simulink model "q_5dof_wand_vr_sphere_collision_atia"  (Simulink 9.1)
settings: Solver=ode1  StartTime=0.0  StopTime=inf  FixedStep=0.001  RelTol=1e-3  EnableMultiTasking=on
values from neighbouring files (symbols this model uses):
  COM = zeros(1,size(V1,2))    [atia_centroid.m]
  fromSI = [1e3 1e3 1e3 180/pi 180/pi]    [setup_wand.m]
  K_CURR = 0.5 * [1 1 -1 -1 1 1]    [setup_wand.m]
  kd = [kd_x kd_y kd_z kd_yaw kd_roll]    [setup_wand.m]
  kp = [kp_x kp_y kp_z kp_yaw kp_roll]    [setup_wand.m]
  vo_c = [0 75 -75] * 1e-3    [setup_wand.m]
  wn_f = 150    [setup_wand.m]
  zeta_f = 1    [setup_wand.m]
undefined symbols (not defined in the file or in its folder): DiscIntNeverNeededParam, HIL, qc_get_step_size, V_CUBE_atia_wand, Visualization
libraries: quarc_library x12
(part 1 of 2)
settings Model: Creator=pmartin  LastModifiedBy=atn227  SimulationMode=external  ExtModeTrigDuration=5000
settings SolverCC: PositivePriorityOrder=on
settings DataIOCC: LimitDataPoints=on  SignalLoggingSaveFormat=ModelDataLogs
settings OptimizationCC: ExpressionDepthLimit=2147483647  LifeSpan=auto
settings DebuggingCC: SolverPrmCheckMsg=warning  FcnCallInpInsideContextMsg=warning  StateNameClashWarn=warning
settings RTWCC: SystemTargetFile=quarc_win64.tlc  TemplateMakefile=quarc_default_tmf  Description=QUARC Win64 Target
settings STFCustomTargetCC: TargetPreCompLibLocation=C:\PROGRA~3\QUARC\lib\2018a\win64\release  ConcurrentExecutionCompliant=on  SystemTargetFile=quarc_win64.tlc
settings GRTTargetCC: TargetPreCompLibLocation=C:\PROGRA~3\QUARC\lib\2018a\win64\release  ParMdlRefBuildCompliant=off  CompOptLevelCompliant=off  MatFileLogging=off  CPPClassGenCompliant=off  UseToolchainInfoCompliant=off  ExtMode=on  ExtModeMexFile=quarc_comm

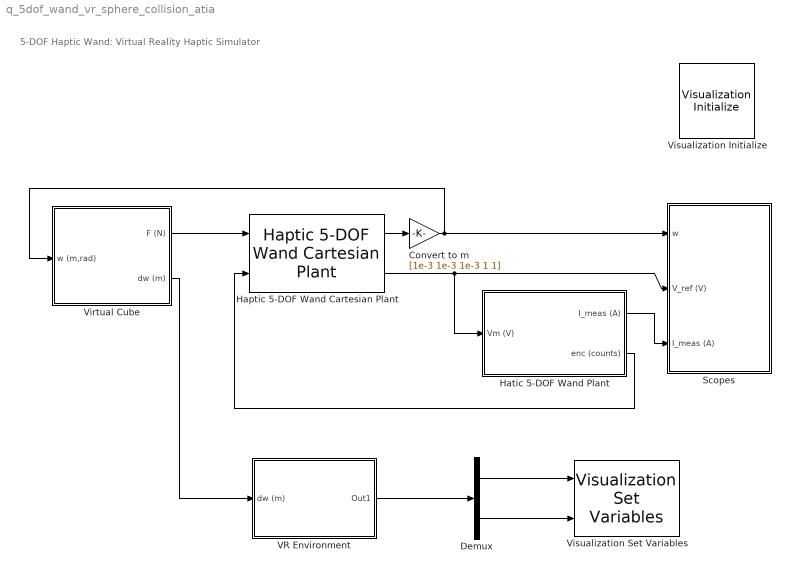
== system q_5dof_wand_vr_sphere_collision_atia ==
  note: 5-DOF Haptic Wand: Virtual Reality Haptic Simulator
  Convert to m : Gain  Gain=[1e-3 1e-3 1e-3 1 1]
  Demux : Demux  Outputs=2
  Haptic 5-DOF Wand Cartesian Plant : quarc_library/Devices/Quanser/Haptics/Pantographs/Haptic 5-DOF Wand/Interfacing/Haptic 5-DOF Wand Cartesian Plant
      settings: SourceProductName=QUARC Targets
  Hatic 5-DOF Wand Plant : Subsystem
  Scopes : Subsystem
  VR Environment : Subsystem
  Virtual Cube : Subsystem
  Visualization Initialize : quarc_library/User Interface/Visualization/Visualization Initialize  object_name=Visualization-1  scene_file=Visualization\5dof_wand_sphere.xml  uri={'normal','';'Configuration','shmem://%m:2';}  apply_uri_to_all_configs=off  server_send_size=1000000  server_receive_size=1000  derive_from_server=on  client_send_size=1000  client_receive_size=1000000  variables=[ 20 21 ]  initial_values=single([ 0 0 0 0 0 0 ])  open_on_start=on  close_on_stop=on
      settings: AttributesFormatString=%<object_name>  SourceProductName=QUARC Targets
  Visualization Set Variables : quarc_library/User Interface/Visualization/Visualization Set Variables  object_name=Visualization-1  offset=[ 3 0 ]  data_type=[ 0 0 ]  length=[ 3 3 ]  sample_time=visualization_get_frame_period  actor_name={'actor.cylinder/Orientation';'actor.cylinder/Position'}
      settings: AttributesFormatString=(%<object_name>)  SourceProductName=QUARC Targets
  wires:
  Virtual Cube/1(F (N)) -> Haptic 5-DOF Wand Cartesian Plant/1
  Virtual Cube/2(dw (m)) -> VR Environment/1(dw (m))
  Haptic 5-DOF Wand Cartesian Plant/2 -> Hatic 5-DOF Wand Plant/1(Vm (V)), Scopes/2(V_ref (V))
  Haptic 5-DOF Wand Cartesian Plant/1 -> Convert to m/1
  Convert to m/1 -> Scopes/1(w), Virtual Cube/1(w (m,rad))
  Hatic 5-DOF Wand Plant/1(I_meas (A)) -> Scopes/3(I_meas (A))
  Hatic 5-DOF Wand Plant/2(enc (counts)) -> Haptic 5-DOF Wand Cartesian Plant/2
  VR Environment/1(Out1) -> Demux/1
  Demux/2 -> Visualization Set Variables/2
  Demux/1 -> Visualization Set Variables/1

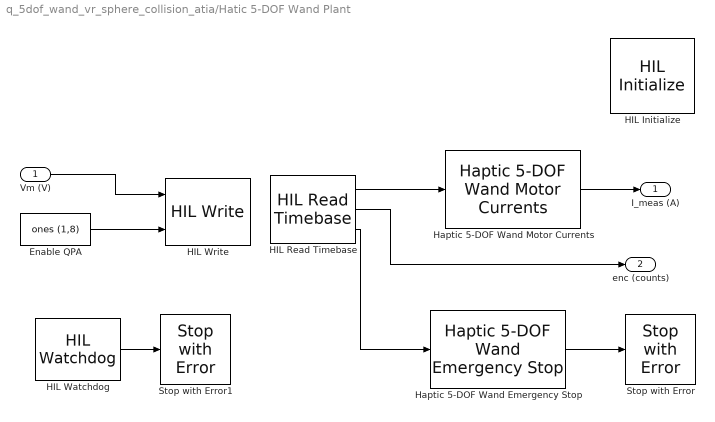
== system q_5dof_wand_vr_sphere_collision_atia/Hatic 5-DOF Wand Plant ==
  Vm (V) : Inport
  Enable QPA : Constant  Value=ones (1,8)
  HIL Initialize : quarc_library/Data Acquisition/Generic/Configuration/HIL Initialize  object_name=HIL-1  board_type=q8  board_number=0  board_options=""  exclusive=off  active=off  hardware_clocks=[0:1]  clock_modes=[0 0]  initial_clock_frequencies=[]  set_clock_params_at_start=on  set_clock_params_at_switch_in=off  set_clock_frequencies_at_start=off  set_clock_frequencies_at_switch_in=off  analog_input_channels=[0:7]  analog_input_configurations=[]  analog_input_maximums=10  analog_input_minimums=-10  set_analog_input_params_at_start=off  set_analog_input_params_at_switch_in=off  analog_output_channels=[0:7]  analog_output_maximums=[10]  analog_output_minimums=[-10]  initial_analog_outputs=[0]  final_analog_outputs=[0]  watchdog_analog_outputs=0  set_analog_output_params_at_start=on  set_analog_output_params_at_switch_in=off  set_analog_outputs_at_start=on  set_analog_outputs_at_switch_in=off  set_analog_outputs_at_terminate=on  set_analog_outputs_at_switch_out=off  set_analog_outputs_on_watchdog=off  digital_input_channels=[]  digital_output_channels=[]  digital_output_configuration=[]  initial_digital_outputs=[1]  final_digital_outputs=[1]  watchdog_digital_outputs=[2]  set_digital_output_params_at_start=off  set_digital_output_params_at_switch_in=off  set_digital_outputs_at_start=on  set_digital_outputs_at_switch_in=off  set_digital_outputs_at_terminate=on  set_digital_outputs_at_switch_out=off  set_digital_outputs_on_watchdog=off  encoder_channels=[0:7]  quadrature=[4]  encoder_filter_frequency=(1/120e-9)/1  initial_encoder_counts=[0]  set_encoder_params_at_start=on  set_encoder_params_at_switch_in=off  set_encoder_counts_at_start=on  set_encoder_counts_at_switch_in=off  pwm_channels=[]  pwm_modes=[0]  pwm_frequency=(1/60e-9)/1024  pwm_configuration=[]  pwm_alignment=[]  pwm_polarity=[]  pwm_leading_deadband=[]  pwm_trailing_deadband=[]  initial_pwm_outputs=[0]  final_pwm_outputs=[0]  watchdog_pwm_outputs=[]  set_pwm_params_at_start=on  set_pwm_params_at_switch_in=off  set_pwm_outputs_at_start=on  set_pwm_outputs_at_switch_in=off  set_pwm_outputs_at_terminate=on  set_pwm_outputs_at_switch_out=off  set_pwm_outputs_on_watchdog=off  other_output_channels=[]  initial_other_outputs=[]  final_other_outputs=[]  watchdog_other_outputs=[]  set_other_outputs_at_start=off  set_other_outputs_at_switch_in=off  set_other_outputs_at_terminate=off  set_other_outputs_at_switch_out=off  set_other_outputs_on_watchdog=off
  HIL Read Timebase : quarc_library/Data Acquisition/Generic/Timebases/HIL Read Timebase  object_name=HIL-1  clock=0  analog_channels=0:5  encoder_channels=[0:5]  digital_channels=[14,30]  other_channels=[]  samples_in_buffer=max(ceil(1/qc_get_step_size), 1)  active=on  vector_output=on  data_type_mode=Inherit via back propagation  encoder_data_type=double  digital_data_type=boolean
  HIL Watchdog : quarc_library/Data Acquisition/Generic/Watchdog/HIL Watchdog  object_name=HIL-1  timeout=qc_get_step_size*10  sample_time=qc_get_step_size  active=off
      settings: AttributesFormatString=(%<object_name>)  SourceProductName=QUARC Targets
  HIL Write : quarc_library/Data Acquisition/Generic/Immediate I//O/HIL Write  object_name=HIL-1  analog_channels=[0:5]  pwm_channels=[]  digital_channels=[0:3 16:19]  other_channels=[]  sample_time=-1  active=off  vector_input=on
  Haptic 5-DOF Wand Emergency Stop : quarc_library/Devices/Quanser/Haptics/Pantographs/Haptic 5-DOF Wand/Interfacing/Haptic 5-DOF Wand Emergency Stop
      settings: SourceProductName=QUARC Targets
  Haptic 5-DOF Wand Motor Currents : quarc_library/Devices/Quanser/Haptics/Pantographs/Haptic 5-DOF Wand/Interfacing/Haptic 5-DOF Wand Motor Currents
      settings: SourceProductName=QUARC Targets
  Stop with Error : quarc_library/Sinks/Error Handling/Stop with Error  message_type=Fixed error message  message=Controller Stopped - Emergency Stop Activated
      settings: AttributesFormatString="\"%<message>\""  SourceProductName=QUARC Targets
  Stop with Error1 : quarc_library/Sinks/Error Handling/Stop with Error  message_type=Fixed error message  message=Stopped by HIL Watchdog - Controller was running too slow
      settings: AttributesFormatString="\"%<message>\""  SourceProductName=QUARC Targets
  I_meas (A) : Outport
  enc (counts) : Outport  Port=2
  wires:
  Haptic 5-DOF Wand Emergency Stop/1 -> Stop with Error/1
  HIL Read Timebase/3 -> Haptic 5-DOF Wand Emergency Stop/1
  Haptic 5-DOF Wand Motor Currents/1 -> I_meas (A)/1
  HIL Read Timebase/2 -> enc (counts)/1
  HIL Read Timebase/1 -> Haptic 5-DOF Wand Motor Currents/1
  Enable QPA/1 -> HIL Write/2
  Vm (V)/1 -> HIL Write/1
  HIL Watchdog/1 -> Stop with Error1/1

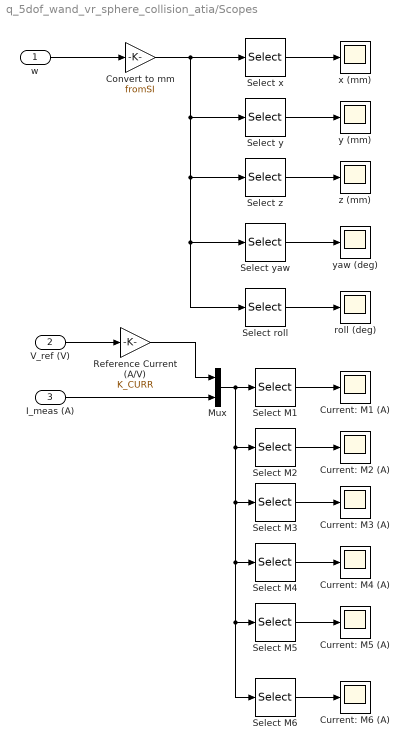
== system q_5dof_wand_vr_sphere_collision_atia/Scopes ==
  w : Inport
  V_ref (V) : Inport  Port=2
  I_meas (A) : Inport  Port=3
  Convert to mm : Gain  Gain=fromSI
  Current: M1 (A) : Scope
  Current: M2 (A) : Scope
  Current: M3 (A) : Scope
  Current: M4 (A) : Scope
  Current: M5 (A) : Scope
  Current: M6 (A) : Scope
  Mux : Mux  Inputs=2
  Reference Current (A/V) : Gain  Gain=K_CURR
  Select M1 : Selector  InputPortWidth=12  IndexOptions=Index vector (dialog)  Indices=[1 7]  OutputSizes=1
  Select M2 : Selector  InputPortWidth=12  IndexOptions=Index vector (dialog)  Indices=[2 8]  OutputSizes=1
  Select M3 : Selector  InputPortWidth=12  IndexOptions=Index vector (dialog)  Indices=[3 9]  OutputSizes=1
  Select M4 : Selector  InputPortWidth=12  IndexOptions=Index vector (dialog)  Indices=[4 10]  OutputSizes=1
  Select M5 : Selector  InputPortWidth=12  IndexOptions=Index vector (dialog)  Indices=[5 11]  OutputSizes=1
  Select M6 : Selector  InputPortWidth=12  IndexOptions=Index vector (dialog)  Indices=[6 12]  OutputSizes=1
  Select roll : Selector  InputPortWidth=5  IndexOptions=Index vector (dialog)  Indices=[5]  OutputSizes=1
  Select x : Selector  InputPortWidth=5  IndexOptions=Index vector (dialog)  Indices=[1]  OutputSizes=1
  Select y : Selector  InputPortWidth=5  IndexOptions=Index vector (dialog)  Indices=2  OutputSizes=1
  Select yaw : Selector  InputPortWidth=5  IndexOptions=Index vector (dialog)  Indices=4  OutputSizes=1
  Select z : Selector  InputPortWidth=5  IndexOptions=Index vector (dialog)  Indices=3  OutputSizes=1
  roll (deg) : Scope
  x (mm) : Scope
  y (mm) : Scope
  yaw (deg) : Scope
  z (mm) : Scope
  wires:
  Convert to mm/1 -> Select x/1, Select y/1, Select roll/1, Select yaw/1, Select z/1
  Select x/1 -> x (mm)/1
  w/1 -> Convert to mm/1
  Select y/1 -> y (mm)/1
  Select z/1 -> z (mm)/1
  Reference Current (A/V)/1 -> Mux/1
  I_meas (A)/1 -> Mux/2
  V_ref (V)/1 -> Reference Current (A/V)/1
  Select yaw/1 -> yaw (deg)/1
  Select roll/1 -> roll (deg)/1
  Mux/1 -> Select M1/1, Select M6/1, Select M5/1, Select M4/1, Select M3/1, Select M2/1
  Select M1/1 -> Current: M1 (A)/1
  Select M2/1 -> Current: M2 (A)/1
  Select M3/1 -> Current: M3 (A)/1
  Select M4/1 -> Current: M4 (A)/1
  Select M5/1 -> Current: M5 (A)/1
  Select M6/1 -> Current: M6 (A)/1

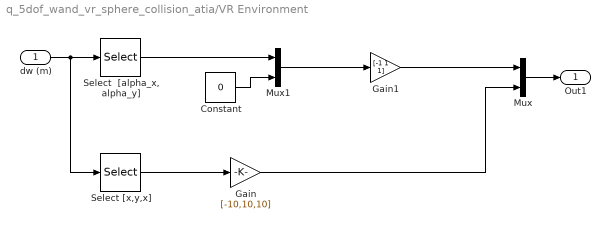
== system q_5dof_wand_vr_sphere_collision_atia/VR Environment ==
  dw (m) : Inport
  Constant : Constant  Value=0
  Gain : Gain  Gain=[-10,10,10]
  Gain1 : Gain  Gain=[-1 1 1]
  Mux : Mux  Inputs=2
  Mux1 : Mux  Inputs=2
  "Select  [alpha_x, alpha_y]" : Selector  InputPortWidth=5  IndexOptions=Index vector (dialog)  Indices=[5,4]  OutputSizes=1
  Select [x,y,x] : Selector  InputPortWidth=5  IndexOptions=Index vector (dialog)  Indices=[2 1 3]  OutputSizes=1
  Out1 : Outport
  wires:
  dw (m)/1 -> "Select  [alpha_x, alpha_y]"/1, Select [x,y,x]/1
  Select [x,y,x]/1 -> Gain/1
  Gain/1 -> Mux/2
  Mux/1 -> Out1/1
  "Select  [alpha_x, alpha_y]"/1 -> Mux1/1
  Mux1/1 -> Gain1/1
  Constant/1 -> Mux1/2
  Gain1/1 -> Mux/1

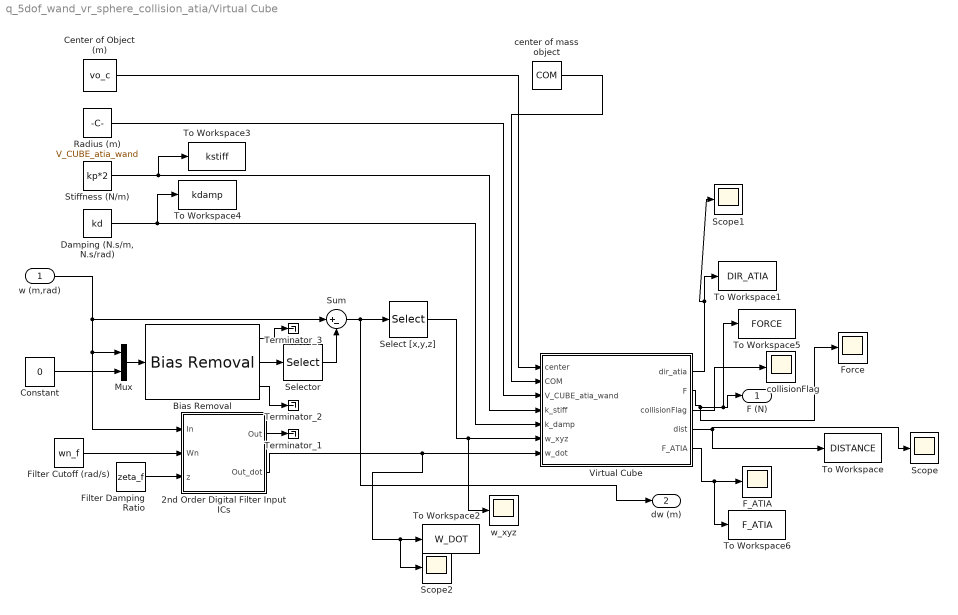
== system q_5dof_wand_vr_sphere_collision_atia/Virtual Cube ==
  w (m,rad) : Inport
  2nd Order Digital Filter Input ICs : Subsystem
  Bias Removal : quarc_library/Discrete/Bias Removal  start_time=0  end_time=qc_get_step_size  switch_id=0  sample_time=qc_get_step_size
      settings: SourceProductName=QUARC Targets
  Center of Object (m) : Constant  Value=vo_c
  Constant : Constant  Value=0
  "Damping (N.s/m, N.s/rad)" : Constant  Value=kd
  F_ATIA : Scope
  Filter Cutoff (rad/s) : Constant  Value=wn_f
  Filter Damping Ratio : Constant  Value=zeta_f
  Force : Scope
  Mux : Mux  Inputs=2
  Radius (m) : Constant  Value=V_CUBE_atia_wand
  Scope : Scope
  Scope1 : Scope
  Scope2 : Scope
  Select [x,y,z] : Selector  InputPortWidth=5  IndexOptions=Index vector (dialog)  Indices=1:3  OutputSizes=1
  Selector : Selector  InputPortWidth=6  IndexOptions=Index vector (dialog)  Indices=1:5  OutputSizes=1
  Stiffness (N/m) : Constant  Value=kp*2
  Sum : Sum  Inputs=|+-
  Terminator_1 : Terminator
  Terminator_2 : Terminator
  Terminator_3 : Terminator
  To Workspace : ToWorkspace  VariableName=DISTANCE  SaveFormat=Timeseries  SampleTime=-1
  To Workspace1 : ToWorkspace  VariableName=DIR_ATIA  SaveFormat=Timeseries  SampleTime=-1
  To Workspace2 : ToWorkspace  VariableName=W_DOT  SaveFormat=Timeseries  SampleTime=-1
      settings: Save2DSignal=2-D array (concatenate along first dimension)
  To Workspace3 : ToWorkspace  VariableName=kstiff  SampleTime=-1
      settings: Save2DSignal=2-D array (concatenate along first dimension)
  To Workspace4 : ToWorkspace  VariableName=kdamp  SampleTime=-1
      settings: Save2DSignal=2-D array (concatenate along first dimension)
  To Workspace5 : ToWorkspace  VariableName=FORCE  SaveFormat=Timeseries  SampleTime=-1
  To Workspace6 : ToWorkspace  VariableName=F_ATIA  SaveFormat=Timeseries  SampleTime=-1
  Virtual Cube : MATLAB Function  TreatAsAtomicUnit=on
  center of mass object : Constant  Value=COM
  collisionFlag : Scope
  w_xyz : Scope
  F (N) : Outport
  dw (m) : Outport  Port=2
  wires:
  Mux/1 -> Bias Removal/1
  Bias Removal/2 -> Selector/1
  Constant/1 -> Mux/2
  w (m,rad)/1 -> Sum/1, Mux/1, 2nd Order Digital Filter Input ICs/1(In)
  Radius (m)/1 -> Virtual Cube/3(V_CUBE_atia_wand)
  Sum/1 -> Select [x,y,z]/1, dw (m)/1
  Selector/1 -> Sum/2
  Center of Object (m)/1 -> Virtual Cube/1(center)
  Stiffness (N/m)/1 -> To Workspace3/1, Virtual Cube/4(k_stiff)
  "Damping (N.s/m, N.s/rad)"/1 -> To Workspace4/1, Virtual Cube/5(k_damp)
  Filter Cutoff (rad/s)/1 -> 2nd Order Digital Filter Input ICs/2(Wn)
  Filter Damping Ratio/1 -> 2nd Order Digital Filter Input ICs/3(z)
  2nd Order Digital Filter Input ICs/2(Out_dot) -> Scope2/1, To Workspace2/1, Virtual Cube/7(w_dot)
  2nd Order Digital Filter Input ICs/1(Out) -> Terminator_1/1
  Select [x,y,z]/1 -> w_xyz/1, Virtual Cube/6(w_xyz)
  Virtual Cube/2(F) -> To Workspace5/1, F (N)/1, Force/1
  Bias Removal/3 -> Terminator_2/1
  Bias Removal/1 -> Terminator_3/1
  Virtual Cube/3(collisionFlag) -> collisionFlag/1
  center of mass object/1 -> Virtual Cube/2(COM)
  Virtual Cube/4(dist) -> Scope/1, To Workspace/1
  Virtual Cube/1(dir_atia) -> Scope1/1, To Workspace1/1
  Virtual Cube/5(F_ATIA) -> To Workspace6/1, F_ATIA/1

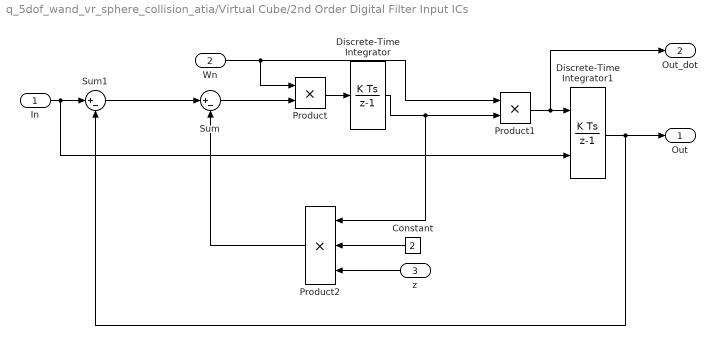
== system q_5dof_wand_vr_sphere_collision_atia/Virtual Cube/2nd Order Digital Filter Input ICs ==
  In : Inport
  Wn : Inport  Port=2
  z : Inport  Port=3
  Constant : Constant  Value=2
  Discrete-Time Integrator : DiscreteIntegrator  Priority=1  SampleTime=qc_get_step_size  ICPrevOutput=DiscIntNeverNeededParam  ICPrevScaledInput=DiscIntNeverNeededParam
  Discrete-Time Integrator1 : DiscreteIntegrator  Priority=1  InitialConditionSource=external  SampleTime=qc_get_step_size  ICPrevOutput=DiscIntNeverNeededParam  ICPrevScaledInput=DiscIntNeverNeededParam
  Product : Product  RndMeth=Zero
  Product1 : Product  RndMeth=Zero
  Product2 : Product  Inputs=3  RndMeth=Zero
  Sum : Sum  Inputs=|+-
  Sum1 : Sum  Inputs=|+-
  Out : Outport
  Out_dot : Outport  Port=2
  wires:
  Product/1 -> Discrete-Time Integrator/1
  Sum/1 -> Product/2
  Wn/1 -> Product/1, Product1/1
  Product1/1 -> Discrete-Time Integrator1/1, Out_dot/1
  Discrete-Time Integrator/1 -> Product1/2, Product2/1
  Discrete-Time Integrator1/1 -> Sum1/2, Out/1
  Sum1/1 -> Sum/1
  In/1 -> Sum1/1, Discrete-Time Integrator1/2
  Product2/1 -> Sum/2
  z/1 -> Product2/3
  Constant/1 -> Product2/2
